simulink model "marsh_velo"  (R2017a)
settings: Solver=VariableStepAuto  StartTime=0.0  StopTime=4  RelTol=1e-3
values from neighbouring files (symbols this model uses):
  Cx = 52.92    [Parameters (2).m]    (also in Parameters.m)
  k2_m = 2.19    [Parameters (2).m]    (also in Parameters.m)
  K_thruster = 2.89    [Parameters (2).m]    (also in Parameters.m)
  lambda11 = 0.6    [Parameters (2).m]    (also in Parameters.m)
  m = 24.7    [Parameters (2).m]    (also in Parameters.m)
  T_thruster = 0.1    [Parameters (2).m]    (also in Parameters.m)
settings Model: Creator=Eugene  LastModifiedBy=Eugene

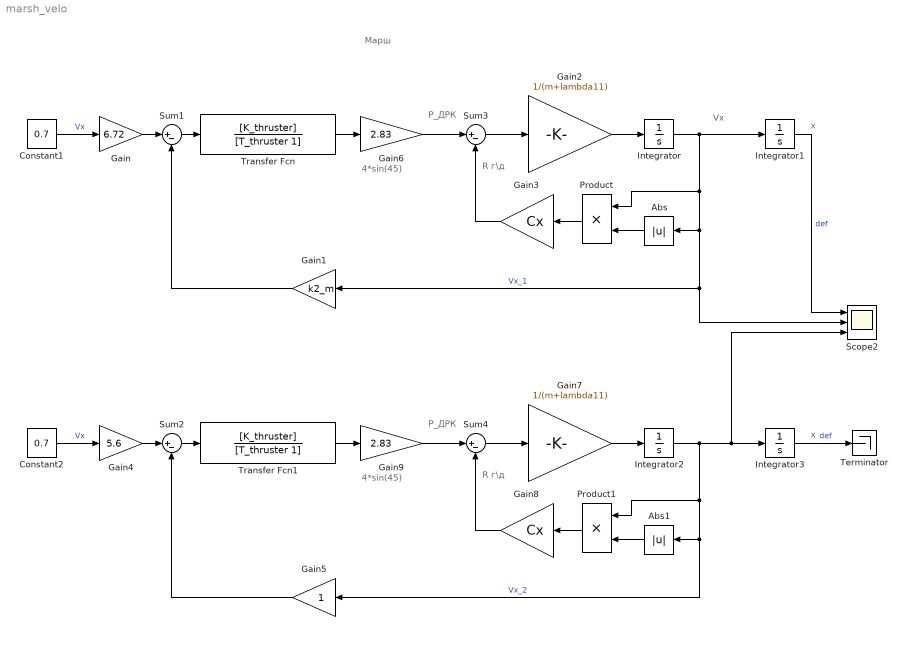
== system marsh_velo ==
  note: R г\д
  note: P_ДРК
  note: 4*sin(45)
  note: Марш
  note: x
  note: Vx
  note: R г\д
  note: P_ДРК
  note: 4*sin(45)
  note: x
  Abs : Abs
  Abs1 : Abs
  Constant1 : Constant  Value=0.7
  Constant2 : Constant  Value=0.7
  Gain : Gain  Gain=6.72
  Gain1 : Gain  Gain=k2_m
  Gain2 : Gain  Gain=1/(m+lambda11)
  Gain3 : Gain  Gain=Cx
  Gain4 : Gain  Gain=5.6
  Gain5 : Gain
  Gain6 : Gain  Gain=2.83
  Gain7 : Gain  Gain=1/(m+lambda11)
  Gain8 : Gain  Gain=Cx
  Gain9 : Gain  Gain=2.83
  Integrator{,1..3} (4 alike) : Integrator
  Product : Product
  Product1 : Product
  Scope2 : Scope  NumInputPorts=3
  Sum{1..4} (4 alike) : Sum  Inputs=|+-
  Terminator : Terminator
  Transfer Fcn : TransferFcn  Numerator=[K_thruster]  Denominator=[T_thruster 1]
  Transfer Fcn1 : TransferFcn  Numerator=[K_thruster]  Denominator=[T_thruster 1]
  wires:
  Constant1/1 -> Gain/1  "Vx"
  Sum1/1 -> Transfer Fcn/1
  Gain2/1 -> Integrator/1
  Abs/1 -> Product/2
  Product/1 -> Gain3/1
  Gain3/1 -> Sum3/2
  Sum3/1 -> Gain2/1
  Transfer Fcn/1 -> Gain6/1
  Gain1/1 -> Sum1/2
  Integrator/1 -> Scope2/2, Gain1/1, Abs/1, Product/1, Integrator1/1  "Vx_1"
  Gain6/1 -> Sum3/1
  Integrator1/1 -> Scope2/1  "def"
  Gain/1 -> Sum1/1
  Gain4/1 -> Sum2/1
  Gain9/1 -> Sum4/1
  Integrator2/1 -> Scope2/3, Integrator3/1, Product1/1, Abs1/1, Gain5/1  "Vx_2"
  Gain5/1 -> Sum2/2
  Transfer Fcn1/1 -> Gain9/1
  Sum4/1 -> Gain7/1
  Gain8/1 -> Sum4/2
  Product1/1 -> Gain8/1
  Abs1/1 -> Product1/2
  Gain7/1 -> Integrator2/1
  Sum2/1 -> Transfer Fcn1/1
  Constant2/1 -> Gain4/1  "Vx"
  Integrator3/1 -> Terminator/1  "def"
